simulink model "ClosedLoop_Cq"  (R2022b)
settings: Solver=VariableStepAuto  StartTime=0.0  StopTime=10.0  RelTol=1e-3
libraries: cstblocks x3
settings Model: Creator=antoninrenoir  LastModifiedBy=emili

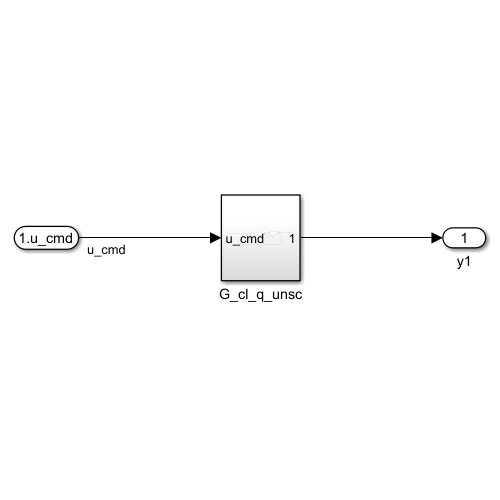
[thumbnail: Simulink's stored preview of the top-level diagram]
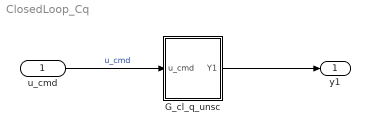
== system ClosedLoop_Cq ==
  u_cmd : Inport
  G_cl_q_unsc : Subsystem
  y1 : Outport
  wires:
  u_cmd/1 -> G_cl_q_unsc/1(u_cmd)  "u_cmd"
  G_cl_q_unsc/1(Y1) -> y1/1

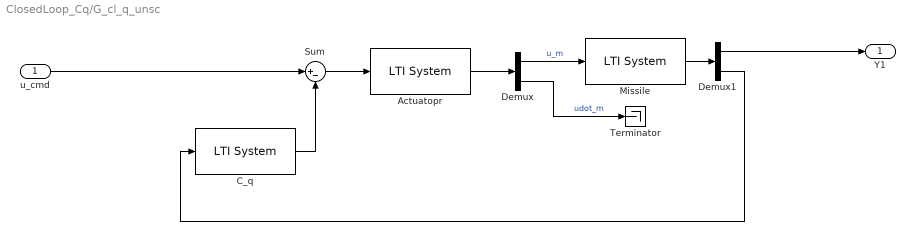
== system ClosedLoop_Cq/G_cl_q_unsc ==
  u_cmd : Inport
  Actuatopr : cstblocks/LTI System  sys=G_a  IC=[]
  C_q : cstblocks/LTI System  sys=C_q  IC=[]
  Demux : Demux  Outputs=2
  Demux1 : Demux  Outputs=2
  Missile : cstblocks/LTI System  sys=G_m  IC=[]
  Sum : Sum  Inputs=|+-
  Terminator : Terminator
  Y1 : Outport
  wires:
  Sum/1 -> Actuatopr/1
  Actuatopr/1 -> Demux/1
  u_cmd/1 -> Sum/1
  Demux1/2 -> C_q/1
  Demux1/1 -> Y1/1
  C_q/1 -> Sum/2
  Missile/1 -> Demux1/1
  Demux/2 -> Terminator/1  "udot_m"
  Demux/1 -> Missile/1  "u_m"
